simulink model "D3"  (R2016b)
settings: Solver=ode45  StartTime=0.0  StopTime=20  RelTol=1e-3
settings Model: Creator=jonathankirchman  LastModifiedBy=jonathankirchman

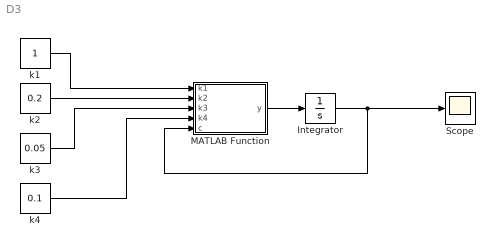
== system D3 ==
  Integrator : Integrator  InitialCondition=[1 0 0]
  MATLAB Function : MATLAB Function  TreatAsAtomicUnit=on
  Scope : Scope
  k1 : Constant
  k2 : Constant  Value=0.2
  k3 : Constant  Value=0.05
  k4 : Constant  Value=0.1
  wires:
  k1/1 -> MATLAB Function/1(k1)
  k2/1 -> MATLAB Function/2(k2)
  k3/1 -> MATLAB Function/3(k3)
  k4/1 -> MATLAB Function/4(k4)
  MATLAB Function/1(y) -> Integrator/1
  Integrator/1 -> Scope/1, MATLAB Function/5(c)

== matlab function D3/MATLAB Function ==
  data: k1 input; y output; k2 input; k3 input; k4 input; c input
function y = D3(k1,k2,k3,k4,c)

y = [-k1*c(1)-k2*c(1)+k3*c(3);...
    2*k1*c(1)-k4*c(2);...
    k2*c(1)-k3*c(3)+k4*c(2)];

end
